simulink model "Test"  (R2023a)
settings: Solver=FixedStepDiscrete  StartTime=0.0  StopTime=5  RelTol=1e-3
libraries: androiduilib x5, androidaudiovideolib x4, androidsensorlib x3
settings Model: Creator=Hitesh  LastModifiedBy=Hitesh
settings OptimizationCC: EnhancedBackFolding=on  PassReuseOutputArgsAs=Individual arguments  ZeroExternalMemoryAtStartup=off  ZeroInternalMemoryAtStartup=off  MaxStackSize=64  OptimizeBlockOrder=speed  DifferentSizesBufferReuse=on  OptimizationCustomize=off  EfficientTunableParamExpr=on
settings DebuggingCC: ParameterTunabilityLossMsg=error
settings HardwareCC: ProdBitPerLong=64  ProdLargestAtomicInteger=LongLong  ProdLargestAtomicFloat=Double  ProdLongLongMode=on  ProdHWDeviceType=ARM Compatible->ARM 64-bit (LP64)  UseEmbeddedCoderFeatures=off  UseSimulinkCoderFeatures=off
settings SFSimCC: MATLABDynamicMemAlloc=off
settings RTWCC: Description=Embedded Coder  SystemTargetFile=ert.tlc  HardwareBoard=Android Device (64bit)  TLCOptions="-aInlineSetEventsForThisBaseRateFcn=TLC_FALSE -aSuppressMultiTaskScheduler=TLC_FALSE  -aRateBasedStepFcn=0"  TemplateMakefile=ert_default_tmf  RTWVerbose=off  Toolchain=Android SDK/NDK Tools
settings CodeAppCC: ForceParamTrailComments=on  IgnoreCustomStorageClasses=off  OperatorAnnotations=on  SimulinkDataObjDesc=on  SFDataObjDesc=on  InsertBlockDesc=on
settings ERTTargetCC: SupportNonInlinedSFcns=on

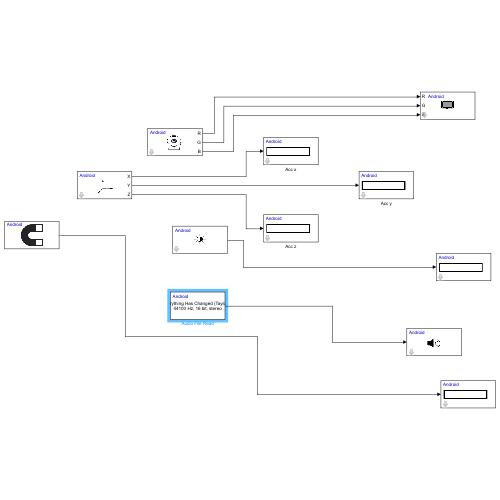
[thumbnail: Simulink's stored preview of the top-level diagram]
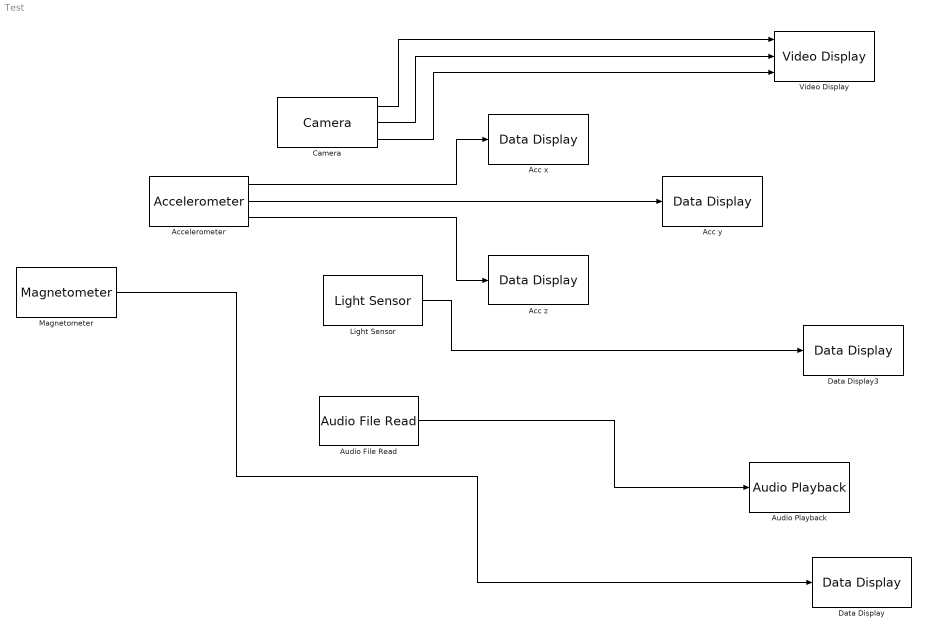
== system Test ==
  Acc x : androiduilib/Data Display  DataDisplayId=Test/Acc_x  Format=Float  Precision=6  SimulateUsing=Code generation  blockPlatform=Android
  Acc y : androiduilib/Data Display  DataDisplayId=Test/Acc_y  Format=Float  Precision=6  SimulateUsing=Code generation  blockPlatform=Android
  Acc z : androiduilib/Data Display  DataDisplayId=Test/Acc_z  Format=Float  Precision=6  SimulateUsing=Code generation  blockPlatform=Android
  Accelerometer : androidsensorlib/Accelerometer  OutputVector=off  SampleTime=0.1  BlockPlatform=Android
  Audio File Read : androidaudiovideolib/Audio File Read  FileName=C:\Users\Hitesh\Music\Taylor Swift - Everything Has Changed (Taylor-'s Version).mp3  FrameSize=4410
  Audio Playback : androidaudiovideolib/Audio Playback  SampleFreq=44100  AudioSamplingFreq=44100  SampleTime=0.1  DeviceStr=0  QueueDuration=0  BlockPlatform=Android
  Camera : androidaudiovideolib/Camera  CameraLocation=Back  CameraResolutions=Back - 2304x1728  Width=2304  Height=1728  SampleTime=0.001  BlockPlatform=Android
  Data Display : androiduilib/Data Display  DataDisplayId=Test/Data_Display  Format=Float  Precision=6  SimulateUsing=Code generation  blockPlatform=Android
  Data Display3 : androiduilib/Data Display  DataDisplayId=Test/Data_Display3  Format=Float  Precision=6  SimulateUsing=Code generation  blockPlatform=Android
  Light Sensor : androidsensorlib/Light Sensor  SampleTime=0.1  BlockPlatform=Android
  Magnetometer : androidsensorlib/Magnetometer  SampleTime=0.1
  Video Display : androidaudiovideolib/Video Display  BlockPlatform=Android
  wires:
  Camera/1 -> Video Display/1
  Camera/2 -> Video Display/2
  Camera/3 -> Video Display/3
  Accelerometer/1 -> Acc x/1
  Accelerometer/2 -> Acc y/1
  Accelerometer/3 -> Acc z/1
  Light Sensor/1 -> Data Display3/1
  Magnetometer/1 -> Data Display/1
  Audio File Read/1 -> Audio Playback/1
